simulink model "bit_manipulation"  (R2023b)
settings: Solver=FixedStepDiscrete  StartTime=0.0  StopTime=10.0  RelTol=1e-3
undefined symbols (not defined in the file or in its folder): bitsperword
libraries: hdlsllib x6
settings Model: DataTypeOverride=Off  Creator=foregan  LastModifiedBy=foregan
settings OptimizationCC: BlockReduction=off  ConditionallyExecuteInputs=off  DefaultParameterBehavior=Inlined  InheritOutputTypeSmallerThanSingle=on
settings DebuggingCC: AlgebraicLoopMsg=error  SingleTaskRateTransMsg=error
settings HardwareCC: ProdBitPerPointer=32  ProdBitPerSizeT=32  ProdBitPerPtrDiffT=32  ProdLargestAtomicFloat=None  ProdIntDivRoundTo=Undefined  ProdEndianess=Unspecified  ProdWordSize=32  ProdHWDeviceType=ASIC/FPGA->ASIC/FPGA  TargetBitPerPointer=64  TargetBitPerSizeT=64  TargetBitPerPtrDiffT=64  TargetLongLongMode=on  TargetIntDivRoundTo=Zero  TargetEndianess=LittleEndian  TargetWordSize=64  TargetHWDeviceType=Custom Processor->MATLAB Host Computer  ProdEqTarget=off

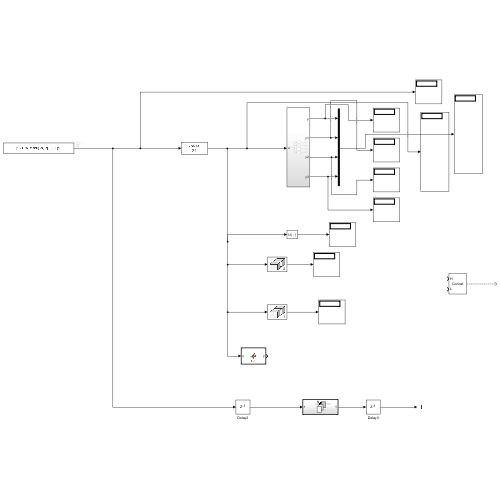
[thumbnail: Simulink's stored preview of the top-level diagram]
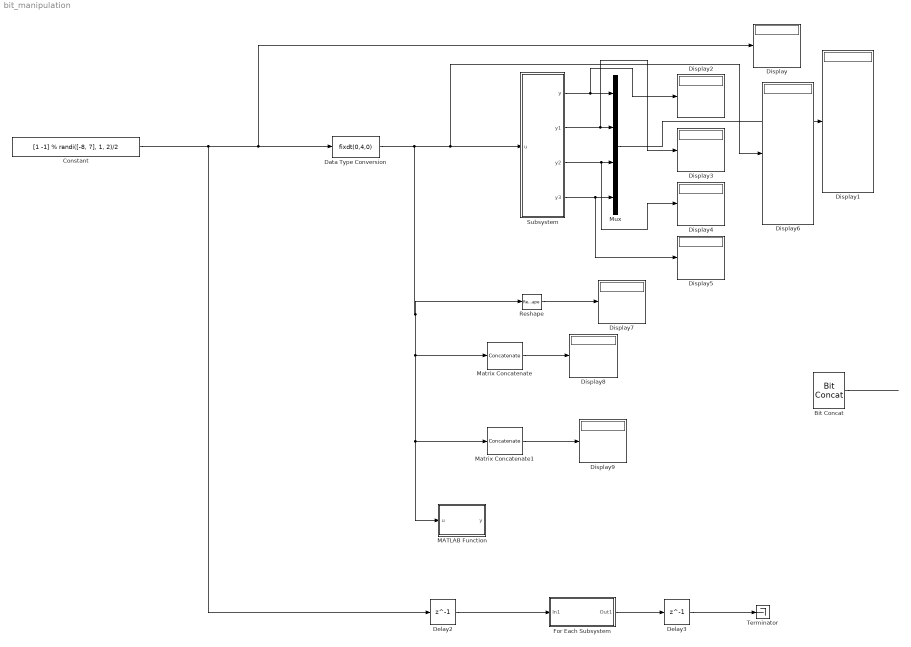
== system bit_manipulation ==
  Bit Concat : hdlsllib/Logic and Bit Operations/Bit Concat  numInputs=2
  Constant : Constant  Value=[1 -1] % randi([-8, 7], 1, 2)/2  OutDataTypeStr=fixdt(1,4,1)  SampleTime=1
  Data Type Conversion : DataTypeConversion  OutDataTypeStr=fixdt(0,4,0)  ConvertRealWorld=Stored Integer (SI)  SaturateOnIntegerOverflow=off  RndMeth=Floor
  Delay2 : Delay  DelayLength=1  InitialCondition=0  UseCircularBuffer=on
  Delay3 : Delay  DelayLength=1  InitialCondition=0  UseCircularBuffer=on
  Display{,1..9} (10 alike) : Display
      Display6 settings: Format=binary (Stored Integer)
  For Each Subsystem : Subsystem  TreatAsAtomicUnit=on
  MATLAB Function : MATLAB Function  TreatAsAtomicUnit=on
  Matrix Concatenate : Concatenate  NumInputs=1  Mode=Multidimensional array  ConcatenateDimension=2
  Matrix Concatenate1 : Concatenate  NumInputs=1  Mode=Multidimensional array
  Mux : Mux
  Reshape : Reshape
  Subsystem : Subsystem
  Terminator : Terminator
  wires:
  Mux/1 -> Display1/1
  Bit Concat/1 -> ?
  Data Type Conversion/1 -> MATLAB Function/1(u), Matrix Concatenate1/1, Matrix Concatenate/1, Reshape/1, Display6/1, Subsystem/1(u)
  Subsystem/1(y) -> Display2/1, Mux/1
  Subsystem/2(y1) -> Display3/1, Mux/2
  Subsystem/3(y2) -> Display4/1, Mux/3
  Subsystem/4(y3) -> Display5/1, Mux/4
  Reshape/1 -> Display7/1
  Matrix Concatenate/1 -> Display8/1
  Matrix Concatenate1/1 -> Display9/1
  Constant/1 -> Delay2/1, Data Type Conversion/1, Display/1
  Delay2/1 -> For Each Subsystem/1(In1)
  For Each Subsystem/1(Out1) -> Delay3/1
  Delay3/1 -> Terminator/1

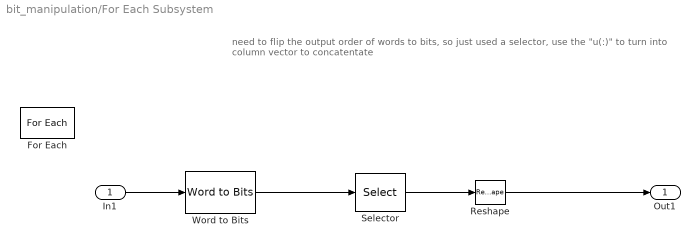
== system bit_manipulation/For Each Subsystem ==
  note: need to flip the output order of words to bits, so just used a selector, use the "u(:)" to turn into column vector to concatentate
  In1 : Inport  Partition=on  PartitionDimension=1  PartitionWidth=1  PartitionOffset=0
  For Each : ForEach  DisableCoverage=on
  Reshape : Reshape
  Selector : Selector  IndexMode=Zero-based  InputPortWidth=bitsperword  IndexOptions=Index vector (dialog)  Indices=[bitsperword-1:-1:0]  OutputSizes=1
  Word to Bits : hdlsllib/Logic and Bit Operations/Word to Bits  maxWordLength=4
  Out1 : Outport  ConcatenationDimension=1
  wires:
  In1/1 -> Word to Bits/1
  Word to Bits/1 -> Selector/1
  Selector/1 -> Reshape/1
  Reshape/1 -> Out1/1

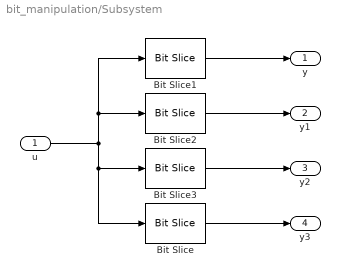
== system bit_manipulation/Subsystem ==
  u : Inport
  Bit Slice : hdlsllib/Logic and Bit Operations/Bit Slice  lidx=0  ridx=0
  Bit Slice1 : hdlsllib/Logic and Bit Operations/Bit Slice  lidx=3  ridx=3
  Bit Slice2 : hdlsllib/Logic and Bit Operations/Bit Slice  lidx=2  ridx=2
  Bit Slice3 : hdlsllib/Logic and Bit Operations/Bit Slice  lidx=1  ridx=1
  y : Outport
  y1 : Outport  Port=2
  y2 : Outport  Port=3
  y3 : Outport  Port=4
  wires:
  u/1 -> Bit Slice1/1, Bit Slice2/1, Bit Slice3/1, Bit Slice/1
  Bit Slice1/1 -> y/1
  Bit Slice3/1 -> y2/1
  Bit Slice2/1 -> y1/1
  Bit Slice/1 -> y3/1

== matlab function bit_manipulation/MATLAB Function ==
  data: u input; y output
function y = fcn(u)
len_u = length(u)
u = u + 1;
y = u
